simulink model "DataCenterStability"  (R2025b)
settings: Solver=daessc  StartTime=0  StopTime=7  FixedStep=5e-5  MaxStep=0.001  RelTol=1e-3
PostLoadFcn:
  | DataCenterParamScan
InitFcn:
  | opFile_ = fullfile(fileparts(which('DataCenterStability')), 'DataCenterStability_SteadyStateOP.mat');
  | if isfile(opFile_)
  |     tmp_ = load(opFile_, 'op');
  |     assignin('base', 'ssOP__', tmp_.op);
  | end
  | warning('off','physmod:common:mf:system:xform:DelayUnsupportedWithOperatingPoint');
  | warning('off','physmod:common:mf:system:xform:TimeUnsupportedWithOperatingPoint');
values from neighbouring files (symbols this model uses):
  baseVoltageDC = ups.Vdc    [DataCenterParamScan.m]
  bessConverterEfficiency = ups.DCBus.converterEff    [DataCenterParamScan.m]
  droopGain = ups.DCBus.droop    [DataCenterParamScan.m]
  filterInductance = ups.inverter.filterInductance    [DataCenterParamScan.m]
  filterInductanceAFE = ups.AFE.filterInductance    [DataCenterParamScan.m]
  filterResistance = ups.inverter.filterResistance    [DataCenterParamScan.m]
  filterResistanceAFE = ups.AFE.filterResistance    [DataCenterParamScan.m]
  frequency = ups.frequency    [DataCenterParamScan.m]
  G1 = 1    [DataCenterParamScan.m]
  G2 = 0    [DataCenterParamScan.m]
  iBatt = ups.batt.iRated    [DataCenterParamScan.m]
  initialMode = ups.batt.initialMode    [DataCenterParamScan.m]
  invKiId = ups.inverter.kiId    [DataCenterParamScan.m]
  invKiVd = ups.inverter.kiVd    [DataCenterParamScan.m]
  invKpId = ups.inverter.kpId    [DataCenterParamScan.m]
  invKpVd = ups.inverter.kpVd    [DataCenterParamScan.m]
  kpDC = ups.DCBus.kpDC    [DataCenterParamScan.m]
  N_pfc = round(N_total * [1/3, 1/3, 1/3])    [DataCenterParamScan.m]    (also in StabilityStudy.m = cfg.Topology.N_pfc)
  plantRating = ups.rating    [DataCenterParamScan.m]
  powerTau = 0.005    [DataCenterParamScan.m]
  rampRate = ups.batt.rampRate    [DataCenterParamScan.m]
  scan = obj.Cfg.GNC    [GNCAnalyzer.m]
  Ts = 5e-5    (= 5e-05)    [DataCenterParamScan.m]
  Vac = ups.Vac    [DataCenterParamScan.m]
  vBattMax = ups.batt.VMax    [DataCenterParamScan.m]
  vBattNom = ups.batt.Vnom    [DataCenterParamScan.m]
  vDCThreshold = ups.DCBus.VThreshold    [DataCenterParamScan.m]
  vGridMin = ups.DCBus.gridThreshold    [DataCenterParamScan.m]
undefined symbols (not defined in the file or in its folder): ctLimitDelayTime, DiscIntNeverNeededParam, ee_sli_rtmsupport, gcbh, itTray, pfc, serverTray, ups
libraries: fl_lib x77, nesl_utility x35, ee_lib x30, simulink x17, eeGeneralControl x14, datacenter_lib x12, eeTransforms x7, slpidlib x4, nesl_utility_internal x4, simulink_extras x3, datacenterCompositeLib x2, eePowerMeasurement x2
(part 4 of 5)

== system DataCenterStability/UPS/Rectifier/PFC Rectifier Controller ==
  VdcRef (V) : Inport
  QRef (pu) : Inport  Port=2
  VdcSens (V) : Inport  Port=3
  VabcSens (pu) : Inport  Port=4
  IabcSens (pu) : Inport  Port=5
  Reset : Inport  Port=6
  Current Controller : Subsystem
  DC Voltage Controller and Current Reference : Subsystem
  PLL : Subsystem
      settings: PortSchema="{\"entries\":[{\"content\":{\"sides\":[{\"content\":{\"connectorIds\":[\"Out1\",\"Out2\",\"Out3\",\"Out4\"]},\"type\":\"ConnectorPlacement.EquallySpacedRectSide\",\"uuid\":\"76485780-20fe-4fcf-8224-69648da6ed2a\"},{\"content\":{\"connectorIds\":[\"In1\"],\"side\":\"RIGHT\"},\"type\":\"ConnectorPlacement.EquallySpacedRectSide\",\"uuid\":\"f19a6390-e634-42c7-8d46-4cd80cbab182\"},{\"content\":{\"side\":\"TOP\"},\"type\":\"ConnectorPlacement.EquallySpacedRectSide\",\"uuid\":\"87682f72-1844-428e-be70-ad7ca3191ee3\"}]},\"type\":\"ConnectorPlacement.EquallySpacedConnector\",\"uuid\":\"f2136b07-48ec-402b-adb3-18c0bac2157c\"}],\"packageUris\":[\"http://schema.mathworks.com/mf0/Connector/R2020b\"],\"version\":\"1.0\"}"
  Rate Transition : RateTransition
  VabcRef (pu) : Outport
  Out Bus Element : Outport  Port=2  PortName=Visualization  Element=pllAngle [rad]
  Out Bus Element1 : Outport  Port=2  PortName=Visualization  Element=pllVmag [pu]
  Out Bus Element2 : Outport  Port=2  PortName=Visualization  Element=Idref [pu]
  Out Bus Element3 : Outport  Port=2  PortName=Visualization  Element=Iqref [pu]
  Out Bus Element5 : Outport  Port=2  PortName=Visualization  Element=IdCntrlError [pu]
  Out Bus Element6 : Outport  Port=2  PortName=Visualization  Element=IqCntrlError [pu]
  wires:
  Current Controller/3(IqCntrlError) -> Out Bus Element6/1
  Current Controller/2(IdCntrlError) -> Out Bus Element5/1
  PLL/1(theta) -> Out Bus Element/1, Current Controller/3(theta)
  Rate Transition/1 -> PLL/1(V)
  DC Voltage Controller and Current Reference/2(iqRef) -> Out Bus Element3/1, Current Controller/2(iqRef)
  DC Voltage Controller and Current Reference/1(idRef) -> Out Bus Element2/1, Current Controller/1(idRef)
  IabcSens (pu)/1 -> Current Controller/6(iabc(PU))
  PLL/3(Vq) -> Current Controller/5(vq)
  PLL/2(Vd) -> Current Controller/4(vd)
  VdcSens (V)/1 -> DC Voltage Controller and Current Reference/4(VdcSens)
  Current Controller/1(vabcRef) -> VabcRef (pu)/1
  PLL/4(mag) -> DC Voltage Controller and Current Reference/2(vPeak), Out Bus Element1/1
  QRef (pu)/1 -> DC Voltage Controller and Current Reference/1(qRef)
  VabcSens (pu)/1 -> Rate Transition/1
  VdcRef (V)/1 -> DC Voltage Controller and Current Reference/3(vdcRef)
  Reset/1 -> Current Controller/7(Reset), DC Voltage Controller and Current Reference/5(Reset)

== system DataCenterStability/UPS/Rectifier/Subsystem ==
  In : Inport
  Constant : Constant  Value=0  OutDataTypeStr=boolean
  Delay : Delay  DelayLength=700  InitialCondition=1  SampleTime=ups.sampleTime
  Detect Decrease : simulink/Logic and Bit Operations/Detect Decrease  vinit=0.0  OutDataTypeStr=boolean
  S-R Flip-Flop1 : simulink_extras/Flip Flops/S-R Flip-Flop  initial_condition=0
  Switch : Switch  Criteria=u2 > Threshold  SaturateOnIntegerOverflow=off  InputSameDT=off
  Out : Outport
  wires:
  In/1 -> Detect Decrease/1, Switch/3, Delay/1
  Switch/1 -> Out/1
  Detect Decrease/1 -> S-R Flip-Flop1/1
  Delay/1 -> Switch/1
  S-R Flip-Flop1/1 -> Switch/2
  Constant/1 -> S-R Flip-Flop1/2

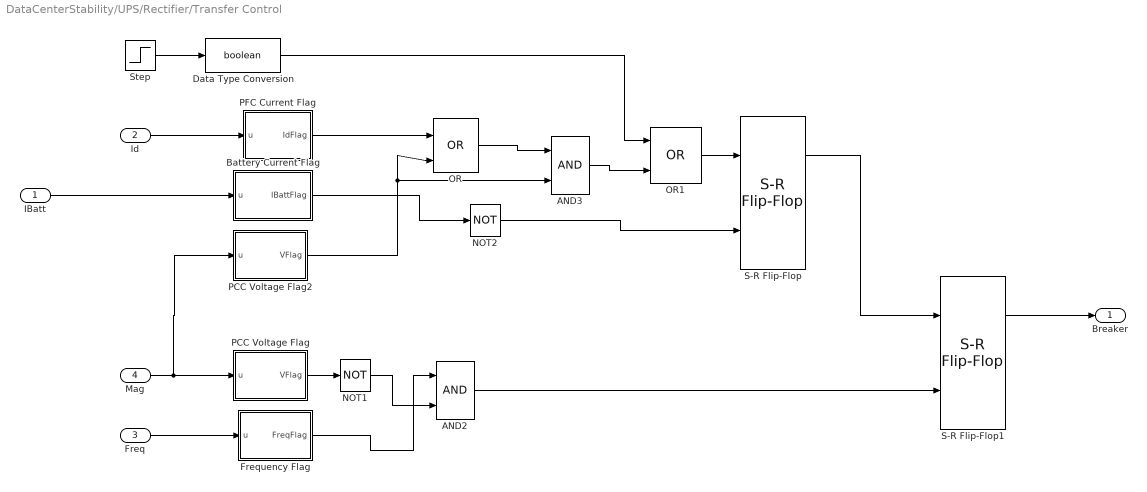
== system DataCenterStability/UPS/Rectifier/Transfer Control ==
  IBatt : Inport
  Id : Inport  Port=2
  Freq : Inport  Port=3
  Mag : Inport  Port=4
  AND2 : Logic  IconShape=distinctive  AllPortsSameDT=off  OutDataTypeStr=boolean
  AND3 : Logic  IconShape=distinctive  AllPortsSameDT=off  OutDataTypeStr=boolean
  Battery Current Flag : Subsystem
  Data Type Conversion : DataTypeConversion  OutDataTypeStr=boolean  SaturateOnIntegerOverflow=off  RndMeth=Floor
  Frequency Flag : Subsystem
  NOT1 : Logic  Operator=NOT  IconShape=distinctive  AllPortsSameDT=off  OutDataTypeStr=boolean
  NOT2 : Logic  Operator=NOT  IconShape=distinctive  AllPortsSameDT=off  OutDataTypeStr=boolean
  OR : Logic  Operator=OR  IconShape=distinctive  AllPortsSameDT=off  OutDataTypeStr=boolean
  OR1 : Logic  Operator=OR  IconShape=distinctive  AllPortsSameDT=off  OutDataTypeStr=boolean
  PCC Voltage Flag : Subsystem
  PCC Voltage Flag2 : Subsystem
  PFC Current Flag : Subsystem
  S-R Flip-Flop : simulink_extras/Flip Flops/S-R Flip-Flop  initial_condition=0
  S-R Flip-Flop1 : simulink_extras/Flip Flops/S-R Flip-Flop  initial_condition=0
  Step : Step  Time=0  SampleTime=0
  Breaker : Outport
  wires:
  PFC Current Flag/1(IdFlag) -> OR/1
  S-R Flip-Flop/1 -> S-R Flip-Flop1/1
  Id/1 -> PFC Current Flag/1(u)
  Mag/1 -> PCC Voltage Flag2/1(u), PCC Voltage Flag/1(u)
  Freq/1 -> Frequency Flag/1(u)
  S-R Flip-Flop1/1 -> Breaker/1
  IBatt/1 -> Battery Current Flag/1(u)
  Frequency Flag/1(FreqFlag) -> AND2/1
  NOT2/1 -> S-R Flip-Flop/2
  Battery Current Flag/1(IBattFlag) -> NOT2/1
  AND2/1 -> S-R Flip-Flop1/2
  OR/1 -> AND3/1
  Step/1 -> Data Type Conversion/1
  AND3/1 -> OR1/2
  Data Type Conversion/1 -> OR1/1
  OR1/1 -> S-R Flip-Flop/1
  PCC Voltage Flag/1(VFlag) -> NOT1/1
  NOT1/1 -> AND2/2
  PCC Voltage Flag2/1(VFlag) -> AND3/2, OR/2

== system DataCenterStability/UPS/DC-Link/BESS/DC-DC Converter Controller ==
  Voref : Inport
  Vo : Inport  Port=2
  vBatt : Inport  Port=3
  iPFC : Inport  Port=4
  iCharge : Inport  Port=5
  iBatt : Inport  Port=6
  vPCC : Inport  Port=7
  Breaker : Inport  Port=8
  Current Reference Generator : Subsystem
  Gain : Gain  Gain=iBatt+4000
  Mode Control : Subsystem
  Saturation : Saturate  UpperLimit=iBatt  LowerLimit=-iBatt
  Simulink-PS Converter : nesl_utility/Simulink-PS Converter  PhysicalDomain=network_engine_domain  SubClassName=ps_input  LeftPortType=input  RightPortType=output  PseudoPeriodic=off  Frequencies=[]  NoiseDistribution=none  NoiseParameters=[]  Unit=1  AffineConversion=off  FilteringAndDerivatives=provide  SimscapeFilterOrder=1  InputFilterTimeConstant=0.001  UdotUserProvided=0
  Terminator1 : Terminator
  mod : PMIOPort  Side=Right
  wires:
  Gain/1 -> Saturation/1
  iPFC/1 -> Mode Control/1(iPFC)
  vBatt/1 -> Mode Control/3(vBatt)
  Current Reference Generator/1(i) -> Gain/1
  Mode Control/1(DischargeFlag) -> Current Reference Generator/2(DischargeFlag)
  Saturation/1 -> Simulink-PS Converter/1
  iBatt/1 -> Mode Control/7(iBatt)
  vPCC/1 -> Mode Control/4(vPCC)
  Breaker/1 -> Mode Control/5(Breaker)
  iCharge/1 -> Mode Control/6(iCharg)
  Vo/1 -> Mode Control/2(Vdc)
  Mode Control/3(iRef) -> Current Reference Generator/4(I)
  Mode Control/5(Mode) -> Terminator1/1
  Voref/1 -> Current Reference Generator/1(VoRef)
  Mode Control/2(vOut) -> Current Reference Generator/3(Vo)
  Mode Control/4(droopMode) -> Current Reference Generator/5(Mode)
  connections:
  mod/RConn1 -- Simulink-PS Converter/RConn1

== system DataCenterStability/UPS/Inverter/Filter & Measurements/ Measurements ==
  V : Inport
  I : Inport  Port=2
  w : Inport  Port=3
  Theta : Inport  Port=4
  Measurement1 : Subsystem
  Measurement2 : Subsystem
  Subsystem : Subsystem
  Out Bus Element : Outport  PortName=VIbus  Element=Vq
  Out Bus Element1 : Outport  PortName=VIbus  Element=Vd
  Out Bus Element2 : Outport  PortName=VIbus  Element=Freq
  Out Bus Element3 : Outport  PortName=VIbus  Element=Theta
  Out Bus Element4 : Outport  PortName=VIbus  Element=Vmag
  Out Bus Element5 : Outport  PortName=VIbus  Element=Iq
  Out Bus Element6 : Outport  PortName=VIbus  Element=Id
  Out Bus Element7 : Outport  PortName=VIbus  Element=Iabc
  Out Bus Element8 : Outport  PortName=VIbus  Element=Vabc
  wires:
  Subsystem/6(Id1) -> Out Bus Element6/1
  Subsystem/7(Iq1) -> Out Bus Element5/1
  Measurement1/1(Vg) -> Subsystem/2(Iabc), Out Bus Element7/1
  I/1 -> Measurement1/1(u)
  Measurement2/1(Vg) -> Subsystem/1(Vabc), Out Bus Element8/1
  Subsystem/4(Vd) -> Out Bus Element1/1
  Subsystem/5(Vq) -> Out Bus Element/1
  V/1 -> Measurement2/1(u)
  w/1 -> Subsystem/3(w)
  Theta/1 -> Subsystem/4(Theta)
  Subsystem/1(mag) -> Out Bus Element4/1
  Subsystem/2(freq) -> Out Bus Element2/1
  Subsystem/3(angle) -> Out Bus Element3/1

== system DataCenterStability/UPS/Inverter/Inverter Controller/Current Limiter ==
  BusElementIn : Inport  PortName=VI  Element=Id
  BusElementIn1 : Inport  PortName=VI  Element=Iq
  Vd : Inport  Port=2
  Vq : Inport  Port=3
  Add : Sum  Inputs=+-
  Add1 : Sum  Inputs=+-
  Current Limiter : Subsystem  Variant=on  VariantControlMode=label  VariantControl=Choice  LabelModeActiveChoice=Virtual Impedance
  VdRef : Outport
  VqRef : Outport  Port=2
  Idmax : Outport  Port=3
  Iqmax : Outport  Port=4
  wires:
  BusElementIn/1 -> Current Limiter/1(Igd)
  BusElementIn1/1 -> Current Limiter/2(Igq)
  Current Limiter/3(Idmax) -> Idmax/1
  Current Limiter/4(Iqmax) -> Iqmax/1
  Current Limiter/1(delVd) -> Add/2
  Vd/1 -> Add/1
  Add1/1 -> VqRef/1
  Current Limiter/2(delVq) -> Add1/2
  Vq/1 -> Add1/1
  Add/1 -> VdRef/1

== system DataCenterStability/UPS/Inverter/Inverter Controller/Droop Control ==
  note: Vs-delV
  Add : Sum  Inputs=+-
  Constant1 : Constant  Value=powerFreq*2*pi
  Constant2 : Constant  Value=0
  Constant3 : Constant
  Constant4 : Constant  Value=0
  Constant5 : Constant  Value=pi/2
  Integrator with Wrapped State (Discrete or Continuous) : eeGeneralControl/Integrator with Wrapped State (Discrete or Continuous)  LabelModeActiveChoice=Discrete  WrappedStateUpperValue=pi  WrappedStateLowerValue=-pi  x0=0  Ts=Ts
  Saturation : Saturate  UpperLimit=1.5  LowerLimit=0.9
  Sum1 : Sum  Inputs=|++
  Vdref : Outport
  Vqref : Outport  Port=2
  omega : Outport  Port=3
  Theta : Outport  Port=4
  wires:
  Constant1/1 -> Integrator with Wrapped State (Discrete or Continuous)/1, omega/1
  Sum1/1 -> Saturation/1  "V"
  Constant5/1 -> Add/2
  Constant3/1 -> Sum1/1
  Saturation/1 -> Vdref/1
  Integrator with Wrapped State (Discrete or Continuous)/1 -> Add/1
  Add/1 -> Theta/1
  Constant4/1 -> Vqref/1
  Constant2/1 -> Sum1/2

== system DataCenterStability/UPS/Inverter/Inverter Controller/VoltageCurrentControl ==
  BusElementIn : Inport  PortName=measure  Element=Vq
  BusElementIn1 : Inport  PortName=measure  Element=Vd
  BusElementIn2 : Inport  PortName=measure  Element=Iq
  BusElementIn3 : Inport  PortName=measure  Element=Id
  Vdref : Inport  Port=2
  Vqref : Inport  Port=3
  Idmax : Inport  Port=4
  Iqmax : Inport  Port=5
  w : Inport  Port=6
  Angle : Inport  Port=7
  Controller : Subsystem
  Modulation Signal : Subsystem
  mabc : Outport
  wires:
  Vdref/1 -> Controller/2(Vdref)
  Controller/1(Vd) -> Modulation Signal/1(Vd)
  Modulation Signal/1(mabc) -> mabc/1
  Controller/2(Vq) -> Modulation Signal/2(Vq)
  w/1 -> Controller/1(Angfreq)
  Angle/1 -> Modulation Signal/3(Angle)
  BusElementIn/1 -> Controller/5(Vsq)
  BusElementIn1/1 -> Controller/4(Vsd)
  BusElementIn2/1 -> Controller/7(Iq)
  BusElementIn3/1 -> Controller/6(Id)
  Vqref/1 -> Controller/3(Vqref)
  Idmax/1 -> Controller/8(IqMax)
  Iqmax/1 -> Controller/9(IdMax)

== system DataCenterStability/UPS/Rectifier/Filter & AC measurements/Current ==
  Isabc : Inport
  Demux : Demux  Outputs=3
  Mux : Mux  Inputs=3
  Unit Delay : UnitDelay  SampleTime=-1
  Iabc : Outport
  wires:
  Mux/1 -> Iabc/1
  Unit Delay/1 -> Demux/1
  Isabc/1 -> Unit Delay/1
  Demux/1 -> Mux/1
  Demux/2 -> Mux/2
  Demux/3 -> Mux/3

== system DataCenterStability/UPS/Rectifier/Filter & AC measurements/PLL ==
  Iabc : Inport
  V : Inport  Port=2
  Constant1 : Constant  Value=pi/2  SampleTime=Ts
  Data Type Conversion Inherited : simulink/Signal Attributes/Data Type Conversion Inherited  ConvertRealWorld=Real World Value  DoSatur=off
  Demux : Demux  Outputs=3
  Park Transform : eeTransforms/Park Transform  AxisAlignment=D-axis  PowerInvariant=off
  "Sinusoidal Measurement (PLL, Three-Phase)" : eeSinusoidalMeasurementV2/Sinusoidal Measurement (PLL, Three-Phase)  InputFilter=on  InputNormalization=off  Kp_LF=ups.AFE.kpPLL  Ki_LF=ups.AFE.kiPLL  F0=frequency  Theta0=0  Ts=Ts
  Sum : Sum  Inputs=|+-
  Terminator : Terminator
  Terminator2 : Terminator
  Id : Outport
  freq : Outport  Port=2
  mag : Outport  Port=3
  wires:
  Data Type Conversion Inherited/1 -> Sum/2
  Constant1/1 -> Data Type Conversion Inherited/2
  V/1 -> "Sinusoidal Measurement (PLL, Three-Phase)"/1
  "Sinusoidal Measurement (PLL, Three-Phase)"/2 -> Sum/1, Data Type Conversion Inherited/1
  Park Transform/1 -> Demux/1
  Demux/3 -> Terminator/1
  Sum/1 -> Park Transform/2
  Demux/1 -> Id/1
  "Sinusoidal Measurement (PLL, Three-Phase)"/1 -> freq/1
  Iabc/1 -> Park Transform/1
  Demux/2 -> Terminator2/1
  "Sinusoidal Measurement (PLL, Three-Phase)"/3 -> mag/1

== system DataCenterStability/UPS/Rectifier/Filter & AC measurements/Voltage ==
  Vsabc : Inport
  Demux1 : Demux  Outputs=3
  Mux1 : Mux  Inputs=3
  Unit Delay : UnitDelay  SampleTime=-1
  Vabc : Outport
  wires:
  Mux1/1 -> Vabc/1
  Unit Delay/1 -> Demux1/1
  Vsabc/1 -> Unit Delay/1
  Demux1/1 -> Mux1/1
  Demux1/2 -> Mux1/2
  Demux1/3 -> Mux1/3

== system DataCenterStability/UPS/Rectifier/PFC Rectifier Controller/Current Controller ==
  idRef : Inport
  iqRef : Inport  Port=2
  theta : Inport  Port=3
  vd : Inport  Port=4
  vq : Inport  Port=5
  iabc(PU) : Inport  Port=6
  Reset : Inport  Port=7
  Demux1 : Demux  Outputs=3
  Id and Iq Controller : Subsystem
  Inverse Park Transform : eeTransforms/Inverse Park Transform  AxisAlignment=D-axis  PowerInvariant=off
  Park Transform : eeTransforms/Park Transform  AxisAlignment=D-axis  PowerInvariant=off
  Saturation : Saturate  UpperLimit=1.5  LowerLimit=-1.5
  Terminator1 : Terminator
  vabcRef : Outport
  IdCntrlError : Outport  Port=2
  IqCntrlError : Outport  Port=3
  wires:
  Id and Iq Controller/2(IdCntrlError) -> IdCntrlError/1
  Id and Iq Controller/3(IqCntrlError) -> IqCntrlError/1
  Id and Iq Controller/1(vdqoRef) -> Inverse Park Transform/1
  vq/1 -> Id and Iq Controller/6(vq)
  Demux1/2 -> Id and Iq Controller/4(iqSens)  "iqSens"
  iqRef/1 -> Id and Iq Controller/2(iqRef)
  Demux1/1 -> Id and Iq Controller/3(IdSens)  "IdSens"
  idRef/1 -> Id and Iq Controller/1(idRef)
  vd/1 -> Id and Iq Controller/5(vd)
  Inverse Park Transform/1 -> Saturation/1
  iabc(PU)/1 -> Park Transform/1
  theta/1 -> Park Transform/2, Inverse Park Transform/2
  Demux1/3 -> Terminator1/1
  Park Transform/1 -> Demux1/1
  Saturation/1 -> vabcRef/1
  Reset/1 -> Id and Iq Controller/7(Reset)

== system DataCenterStability/UPS/Rectifier/PFC Rectifier Controller/DC Voltage Controller and Current Reference ==
  qRef : Inport
  vPeak : Inport  Port=2
  vdcRef : Inport  Port=3
  VdcSens : Inport  Port=4
  Reset : Inport  Port=5
  Constant : Constant  SampleTime=Ts
  Data Type Conversion Inherited : simulink/Signal Attributes/Data Type Conversion Inherited  ConvertRealWorld=Real World Value  DoSatur=off
  Gain : Gain  Gain=-1
  Iq Reference : Subsystem
  Switch : Switch  Criteria=u2 > Threshold  SaturateOnIntegerOverflow=off  InputSameDT=off
  Voltage Controller : Subsystem
  idRef : Outport
  iqRef : Outport  Port=2
  wires:
  Constant/1 -> Data Type Conversion Inherited/2
  Data Type Conversion Inherited/1 -> Switch/3
  Gain/1 -> iqRef/1
  qRef/1 -> Iq Reference/2(Q_ref)
  Voltage Controller/1(Id) -> idRef/1
  vdcRef/1 -> Voltage Controller/1(Vdcref)
  VdcSens/1 -> Voltage Controller/2(Vdcmeas)
  Iq Reference/1(iq_ref) -> Gain/1
  vPeak/1 -> Switch/2, Switch/1, Data Type Conversion Inherited/1
  Switch/1 -> Iq Reference/1(V_mag)
  Reset/1 -> Voltage Controller/3(Reset)

== system DataCenterStability/UPS/Rectifier/PFC Rectifier Controller/PLL ==
  V : Inport
  Constant1 : Constant  Value=pi/2  SampleTime=Ts
  Data Type Conversion Inherited : simulink/Signal Attributes/Data Type Conversion Inherited  ConvertRealWorld=Real World Value  DoSatur=off
  Demux : Demux  Outputs=3
  Park Transform : eeTransforms/Park Transform  AxisAlignment=D-axis  PowerInvariant=off
  "Sinusoidal Measurement (PLL, Three-Phase)" : eeSinusoidalMeasurementV2/Sinusoidal Measurement (PLL, Three-Phase)  InputFilter=on  InputNormalization=off  Kp_LF=KpPLL  Ki_LF=KiPLL  F0=Freq  Theta0=0  Ts=Ts
  Sum : Sum  Inputs=|+-
  Terminator : Terminator
  Terminator1 : Terminator
  theta : Outport
  Vd : Outport  Port=2
  Vq : Outport  Port=3
  mag : Outport  Port=4
  wires:
  Data Type Conversion Inherited/1 -> Sum/2
  Constant1/1 -> Data Type Conversion Inherited/2
  V/1 -> Park Transform/1, "Sinusoidal Measurement (PLL, Three-Phase)"/1
  "Sinusoidal Measurement (PLL, Three-Phase)"/2 -> Sum/1, Data Type Conversion Inherited/1
  Park Transform/1 -> Demux/1
  Demux/3 -> Terminator/1
  "Sinusoidal Measurement (PLL, Three-Phase)"/3 -> mag/1
  Sum/1 -> Park Transform/2, theta/1
  Demux/2 -> Vq/1
  Demux/1 -> Vd/1
  "Sinusoidal Measurement (PLL, Three-Phase)"/1 -> Terminator1/1

== system DataCenterStability/UPS/Rectifier/Transfer Control/Battery Current Flag ==
  u : Inport
  AND : Logic  IconShape=distinctive  AllPortsSameDT=off  OutDataTypeStr=boolean
  Compare To Constant : simulink/Logic and Bit Operations/Compare To Constant  relop=>=  const=0.04  OutDataTypeStr=boolean
  Compare To Constant1 : simulink/Logic and Bit Operations/Compare To Constant  relop=<=  const=-10  OutDataTypeStr=boolean
  Data Type Conversion : DataTypeConversion  SaturateOnIntegerOverflow=off  RndMeth=Floor
  Data Type Conversion1 : DataTypeConversion  OutDataTypeStr=double  SaturateOnIntegerOverflow=off  RndMeth=Floor
  Discrete-Time Integrator : DiscreteIntegrator  IntegratorMethod=Integration: Backward Euler  ExternalReset=falling  SampleTime=ups.sampleTime  LimitOutput=on  UpperSaturationLimit=0.04  LowerSaturationLimit=0  ICPrevOutput=DiscIntNeverNeededParam  ICPrevScaledInput=DiscIntNeverNeededParam
  Scope : Scope  NumInputPorts=2
      settings: ActiveDisplayYMinimum=-1  ActiveDisplayYMaximum=1  DataLoggingVariableName=ScopeData51
  Scope1 : Scope
      settings: ActiveDisplayYMinimum=-1  ActiveDisplayYMaximum=1  DataLoggingVariableName=ScopeData52
  Scope2 : Scope
      settings: ActiveDisplayYMinimum=-1  ActiveDisplayYMaximum=1  DataLoggingVariableName=ScopeData54
  IBattFlag : Outport
  wires:
  AND/1 -> Data Type Conversion/1
  Compare To Constant1/1 -> Data Type Conversion1/1
  Compare To Constant/1 -> AND/2
  u/1 -> Scope2/1, Compare To Constant1/1
  Discrete-Time Integrator/1 -> Scope/2, Compare To Constant/1
  Data Type Conversion/1 -> Scope1/1, IBattFlag/1
  Data Type Conversion1/1 -> Discrete-Time Integrator/1, Scope/1, AND/1, Discrete-Time Integrator/2

== system DataCenterStability/UPS/Rectifier/Transfer Control/Frequency Flag ==
  u : Inport
  AND : Logic  IconShape=distinctive  AllPortsSameDT=off  OutDataTypeStr=boolean
  Abs : Abs  SaturateOnIntegerOverflow=off
  Add : Sum  Inputs=+-
  Compare To Constant : simulink/Logic and Bit Operations/Compare To Constant  relop=>  const=0.5  OutDataTypeStr=boolean
  Compare To Constant1 : simulink/Logic and Bit Operations/Compare To Constant  relop=<=  const=0.01*frequency  OutDataTypeStr=boolean
  Constant : Constant  Value=frequency
  Data Type Conversion : DataTypeConversion  SaturateOnIntegerOverflow=off  RndMeth=Floor
  Data Type Conversion1 : DataTypeConversion  OutDataTypeStr=double  SaturateOnIntegerOverflow=off  RndMeth=Floor
  Discrete-Time Integrator : DiscreteIntegrator  IntegratorMethod=Integration: Backward Euler  ExternalReset=falling  SampleTime=ups.sampleTime  LimitOutput=on  UpperSaturationLimit=0.6  LowerSaturationLimit=0  ICPrevOutput=DiscIntNeverNeededParam  ICPrevScaledInput=DiscIntNeverNeededParam
  FreqFlag : Outport
  wires:
  AND/1 -> Data Type Conversion/1
  Compare To Constant/1 -> AND/2
  Discrete-Time Integrator/1 -> Compare To Constant/1
  Data Type Conversion/1 -> FreqFlag/1
  Data Type Conversion1/1 -> Discrete-Time Integrator/1, AND/1, Discrete-Time Integrator/2
  u/1 -> Add/1
  Constant/1 -> Add/2
  Add/1 -> Abs/1
  Abs/1 -> Compare To Constant1/1
  Compare To Constant1/1 -> Data Type Conversion1/1

== system DataCenterStability/UPS/Rectifier/Transfer Control/PCC Voltage Flag ==
  u : Inport
  AND : Logic  IconShape=distinctive  AllPortsSameDT=off  OutDataTypeStr=boolean
  Abs : Abs  SaturateOnIntegerOverflow=off
  Add : Sum  Inputs=+-
  Compare To Constant : simulink/Logic and Bit Operations/Compare To Constant  relop=>  const=0.2  OutDataTypeStr=boolean
  Compare To Constant1 : simulink/Logic and Bit Operations/Compare To Constant  relop=>=  const=0.1  OutDataTypeStr=boolean
  Constant : Constant
  Data Type Conversion : DataTypeConversion  SaturateOnIntegerOverflow=off  RndMeth=Floor
  Data Type Conversion1 : DataTypeConversion  OutDataTypeStr=double  SaturateOnIntegerOverflow=off  RndMeth=Floor
  Discrete-Time Integrator : DiscreteIntegrator  IntegratorMethod=Integration: Backward Euler  ExternalReset=falling  SampleTime=ups.sampleTime  LimitOutput=on  UpperSaturationLimit=0.6  LowerSaturationLimit=0  ICPrevOutput=DiscIntNeverNeededParam  ICPrevScaledInput=DiscIntNeverNeededParam
  VFlag : Outport
  wires:
  AND/1 -> Data Type Conversion/1
  Compare To Constant/1 -> AND/2
  Discrete-Time Integrator/1 -> Compare To Constant/1
  Data Type Conversion/1 -> VFlag/1
  Data Type Conversion1/1 -> Discrete-Time Integrator/1, AND/1, Discrete-Time Integrator/2
  u/1 -> Add/1
  Constant/1 -> Add/2
  Add/1 -> Abs/1
  Compare To Constant1/1 -> Data Type Conversion1/1
  Abs/1 -> Compare To Constant1/1

== system DataCenterStability/UPS/Rectifier/Transfer Control/PCC Voltage Flag2 ==
  u : Inport
  AND : Logic  IconShape=distinctive  AllPortsSameDT=off  OutDataTypeStr=boolean
  Abs : Abs  SaturateOnIntegerOverflow=off
  Add : Sum  Inputs=+-
  Compare To Constant : simulink/Logic and Bit Operations/Compare To Constant  relop=>  const=0.15  OutDataTypeStr=boolean
  Compare To Constant1 : simulink/Logic and Bit Operations/Compare To Constant  relop=>=  const=0.9  OutDataTypeStr=boolean
  Constant : Constant
  Data Type Conversion : DataTypeConversion  SaturateOnIntegerOverflow=off  RndMeth=Floor
  Data Type Conversion1 : DataTypeConversion  OutDataTypeStr=double  SaturateOnIntegerOverflow=off  RndMeth=Floor
  Discrete-Time Integrator : DiscreteIntegrator  IntegratorMethod=Integration: Backward Euler  ExternalReset=falling  SampleTime=ups.sampleTime  LimitOutput=on  UpperSaturationLimit=4  LowerSaturationLimit=0  ICPrevOutput=DiscIntNeverNeededParam  ICPrevScaledInput=DiscIntNeverNeededParam
  VFlag : Outport
  wires:
  AND/1 -> Data Type Conversion/1
  Compare To Constant/1 -> AND/2
  Discrete-Time Integrator/1 -> Compare To Constant/1
  Data Type Conversion/1 -> VFlag/1
  Data Type Conversion1/1 -> Discrete-Time Integrator/1, AND/1, Discrete-Time Integrator/2
  u/1 -> Add/1
  Constant/1 -> Add/2
  Add/1 -> Abs/1
  Compare To Constant1/1 -> Data Type Conversion1/1
  Abs/1 -> Compare To Constant1/1

== system DataCenterStability/UPS/Rectifier/Transfer Control/PFC Current Flag ==
  u : Inport
  AND : Logic  IconShape=distinctive  AllPortsSameDT=off  OutDataTypeStr=boolean
  Compare To Constant : simulink/Logic and Bit Operations/Compare To Constant  relop=>  const=0.02  OutDataTypeStr=boolean
  Compare To Constant1 : simulink/Logic and Bit Operations/Compare To Constant  relop=<=  const=0.01  OutDataTypeStr=boolean
  Data Type Conversion : DataTypeConversion  SaturateOnIntegerOverflow=off  RndMeth=Floor
  Data Type Conversion1 : DataTypeConversion  OutDataTypeStr=double  SaturateOnIntegerOverflow=off  RndMeth=Floor
  Discrete-Time Integrator : DiscreteIntegrator  IntegratorMethod=Integration: Backward Euler  ExternalReset=falling  SampleTime=ups.sampleTime  LimitOutput=on  UpperSaturationLimit=0.04  LowerSaturationLimit=0  ICPrevOutput=DiscIntNeverNeededParam  ICPrevScaledInput=DiscIntNeverNeededParam
  Scope : Scope  NumInputPorts=2
      settings: ActiveDisplayYMinimum=-1  ActiveDisplayYMaximum=1  DataLoggingVariableName=ScopeData49
  Scope1 : Scope
      settings: ActiveDisplayYMinimum=-1  ActiveDisplayYMaximum=1  DataLoggingVariableName=ScopeData50
  IdFlag : Outport
  wires:
  AND/1 -> Data Type Conversion/1
  Compare To Constant1/1 -> Data Type Conversion1/1
  Compare To Constant/1 -> Scope/2, AND/2
  u/1 -> Compare To Constant1/1
  Discrete-Time Integrator/1 -> Scope1/1, Compare To Constant/1
  Data Type Conversion/1 -> IdFlag/1
  Data Type Conversion1/1 -> Scope/1, Discrete-Time Integrator/1, AND/1, Discrete-Time Integrator/2

== system DataCenterStability/UPS/DC-Link/BESS/DC-DC Converter Controller/Current Reference Generator ==
  VoRef : Inport
  DischargeFlag : Inport  Port=2
  Vo : Inport  Port=3
  I : Inport  Port=4
  Mode : Inport  Port=5
  Add : Sum  Inputs=-+
  Gain : Gain  Gain=droopGain
  Low-Pass Filter (Discrete or Continuous) : eeGeneralControl/Low-Pass Filter (Discrete or Continuous)  K=1  T=0.001  B=inf  A=-inf  init_option=Inherited from block input  x0=0  Ts=-1
  PID Controller : slpidlib/PID Controller  Controller=PI  Form=Parallel  TimeDomain=Discrete-time  UseExternalTs=off  SampleTime=-1  IntegratorMethod=Forward Euler  FilterMethod=Forward Euler  ControllerParametersSource=internal  P=kpDC%500  I=kiDC%500  UseKiTs=off  D=0  UseExternalDerivativeSource=off  N=100  UseFilter=on  TunerSelectOption=Transfer Function Based (PID Tuner App)  InitialConditionSource=internal  InitialConditionForIntegrator=0  InitialConditionForFilter=0  DifferentiatorICPrevScaledInput=0  ExternalReset=rising  TrackingMode=off  Kt=1  LimitOutput=on  SatLimitsSource=internal  UpperSaturationLimit=0  LowerSaturationLimit=-5  LinearizeAsGain=on  AntiWindupMode=clamping  Kb=1  LimitIntegrator=off  UpperIntegratorSaturationLimit=4  LowerIntegratorSaturationLimit=-4  POutMin=[]  POutMax=[]  IOutMin=[]  IOutMax=[]  DOutMin=[]  DOutMax=[]  NOutMin=[]  NOutMax=[]  SumOutMin=[]  SumOutMax=[]  SaturationOutMin=[]  SaturationOutMax=[]  PParamMin=[]  PParamMax=[]  IParamMin=[]  IParamMax=[]  DParamMin=[]  DParamMax=[]  NParamMin=[]  NParamMax=[]  KbParamMin=[]  KbParamMax=[]  KtParamMin=[]  KtParamMax=[]  KbOutMin=[]  KbOutMax=[]  KtOutMin=[]  KtOutMax=[]  IntegratorOutMin=[]  IntegratorOutMax=[]  FilterOutMin=[]  FilterOutMax=[]  SumI1OutMin=[]  SumI1OutMax=[]  SumI2OutMin=[]  SumI2OutMax=[]  SumI3OutMin=[]  SumI3OutMax=[]  SumI4OutMin=[]  SumI4OutMax=[]  SumDOutMin=[]  SumDOutMax=[]  DifferentiatorOutMin=[]  DifferentiatorOutMax=[]  FilterDiffOutCoefMin=[]  FilterDiffOutCoefMax=[]  ReciprocalOutMin=[]  ReciprocalOutMax=[]  SumDenOutMin=[]  SumDenOutMax=[]  SumNumOutMin=[]  SumNumOutMax=[]  DivideOutMin=[]  DivideOutMax=[]  UdiffTsProdOutMin=[]  UdiffTsProdOutMax=[]  NTsProdOutMin=[]  NTsProdOutMax=[]  UintegralTsProdOutMin=[]  UintegralTsProdOutMax=[]  UngainTsProdOutMin=[]  UngainTsProdOutMax=[]  ClampingZeroOutDataTypeStr=Inherit: Inherit via back propagation  ClampingZeroOutMin=[]  ClampingZeroOutMax=[]  FilterDenConstantOutDataTypeStr=Inherit: Inherit via back propagation  FilterDenConstantOutMin=[]  FilterDenConstantOutMax=[]  PCopyOutDataTypeStr=Inherit: Inherit via back propagation  PCopyOutMin=[]  PCopyOutMax=[]  NCopyOutDataTypeStr=Inherit: Inherit via back propagation  NCopyOutMin=[]  NCopyOutMax=[]  IntegratorContinuousStateAttributes=''  IntegratorStateMustResolveToSignalObject=off  IntegratorRTWStateStorageClass=Auto  FilterContinuousStateAttributes=''  FilterStateMustResolveToSignalObject=off  FilterRTWStateStorageClass=Auto  ParallelPVariant=InternalParameters  IdealPVariant=Disabled  IVariant=InternalParameters  DVariant=Disabled  IntegratorVariant=Discrete  SatVariant=Enabled  AWVariant=DiscClampingParallel  PCopyVariant=Disabled  TRVariant=Disabled  FdbkBlocksVariant=Forward  IdealPFdbkVariant=Disabled  SatFdbkVariant=Disabled  DerivativeFilterVariant=Disabled  NVariant=Disabled  NCopyVariant=Disabled_SignalSpec  FilterICVariant=Disabled  IntegratorICVariant=InternalICs  ExternalResetVariant=ExternalReset  TRSumVariant=Passthrough  SumFdbkVariant=Disabled  SumVariant=Sum_PI  TsampFilterVariant=InternalTs  TsampNgainVariant=Passthrough  TsampIntegralVariant=Disabled_SignalSpec  ExternalSaturationOutDataTypeStr=Inherit: Same as second input  DerivativeSourceVariant=Disabled  PreIntVariant=InternalPreInt
  Saturation1 : Saturate  UpperLimit=0  LowerLimit=-10
  Switch1 : Switch  Criteria=u2 > Threshold  SaturateOnIntegerOverflow=off  InputSameDT=off
  Switch3 : Switch  Criteria=u2 > Threshold  SaturateOnIntegerOverflow=off  InputSameDT=off
  i : Outport  VectorParamsAs1DForOutWhenUnconnected=off
  wires:
  Switch1/1 -> Low-Pass Filter (Discrete or Continuous)/1
  Low-Pass Filter (Discrete or Continuous)/1 -> i/1
  Gain/1 -> Saturation1/1
  Switch3/1 -> Switch1/1
  Add/1 -> PID Controller/1, Gain/1
  VoRef/1 -> Add/1
  Vo/1 -> Add/2
  DischargeFlag/1 -> PID Controller/2, Switch1/2
  Mode/1 -> Switch3/2
  Saturation1/1 -> Switch3/1
  PID Controller/1 -> Switch3/3
  I/1 -> Switch1/3

== system DataCenterStability/UPS/DC-Link/BESS/DC-DC Converter Controller/Mode Control ==
  iPFC : Inport
  Vdc : Inport  Port=2
  vBatt : Inport  Port=3
  vPCC : Inport  Port=4
  Breaker : Inport  Port=5
  iCharg : Inport  Port=6
  iBatt : Inport  Port=7
  BMS : Stateflow chart  TreatAsAtomicUnit=on  mask(Microgrid Transition and Dispatch Control){VMaxBatt=vBattMax, VdcRated=baseVoltageDC, iThreshold=vGridMin, iBattTh=10, vThreshold=0.9, VMaxDC=vDCThreshold, VBattNom=vBattMax, initialMode=initialMode}
      mask prompts: VMaxBatt "Maximum Battery Voltage (V)"; VdcRated "Rated DC bus voltage (V)"; iThreshold "Threshold mains current (A)"; iBattTh "Threshold battery current (A)"; vThreshold "Threshold mains voltage (V)"; VMaxDC "Threshold DC Bus Voltage (V)"; VBattNom "Battery nominal voltage (V)"; initialMode "Initial Operating Mode"
      mask help: This subsystem implements the transitions and the corresponding dispatch functions in the microgrid
  Compare To Constant : simulink/Logic and Bit Operations/Compare To Constant  relop===  const=4  OutDataTypeStr=boolean
  Constant : Constant  Value=0.98  OutDataTypeStr=double
  DischargeFlag : Outport
  vOut : Outport  Port=2
  iRef : Outport  Port=3
  droopMode : Outport  Port=4
  Mode : Outport  Port=5
  wires:
  iPFC/1 -> BMS/1(iPFC)
  Vdc/1 -> BMS/2(Vdc)
  vBatt/1 -> BMS/3(VBatt)
  Compare To Constant/1 -> DischargeFlag/1
  Constant/1 -> BMS/4(SOC)
  Breaker/1 -> BMS/5(breakerStatus)
  BMS/1(mode) -> Compare To Constant/1, Mode/1
  vPCC/1 -> BMS/6(VPCC)
  iCharg/1 -> BMS/7(iCharg)
  BMS/3(vOut) -> vOut/1
  BMS/2(iRef) -> iRef/1
  iBatt/1 -> BMS/8(iBatt)
  BMS/4(droopMode) -> droopMode/1

== system DataCenterStability/UPS/Inverter/Filter & Measurements/ Measurements/Measurement1 ==
  u : Inport
  Lead-Lag (Discrete or Continuous) : eeGeneralControl/Lead-Lag (Discrete or Continuous)  T1=0  T2=1e-3  B=inf  A=-inf  init_option=Inherited from block input  x0=0  Ts=Ts
  Vg : Outport
  wires:
  u/1 -> Lead-Lag (Discrete or Continuous)/1
  Lead-Lag (Discrete or Continuous)/1 -> Vg/1

== system DataCenterStability/UPS/Inverter/Filter & Measurements/ Measurements/Measurement2 ==
  u : Inport
  Lead-Lag (Discrete or Continuous) : eeGeneralControl/Lead-Lag (Discrete or Continuous)  T1=0  T2=1e-3  B=inf  A=-inf  init_option=Inherited from block input  x0=0  Ts=Ts
  Vg : Outport
  wires:
  u/1 -> Lead-Lag (Discrete or Continuous)/1
  Lead-Lag (Discrete or Continuous)/1 -> Vg/1

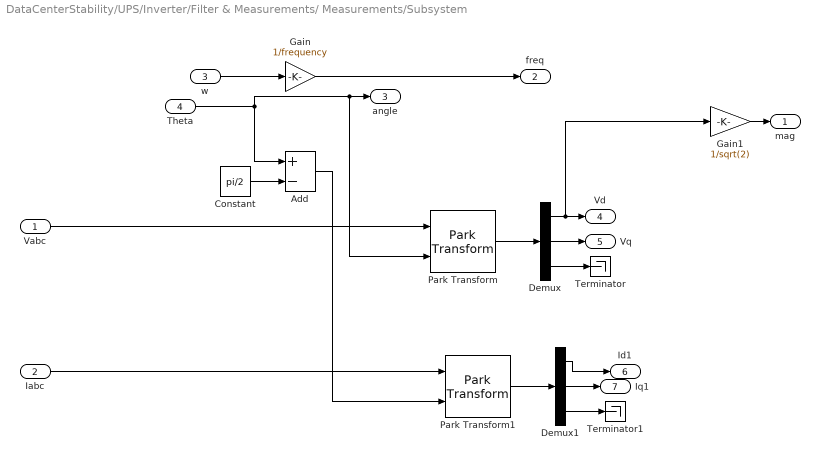
== system DataCenterStability/UPS/Inverter/Filter & Measurements/ Measurements/Subsystem ==
  Vabc : Inport
  Iabc : Inport  Port=2
  w : Inport  Port=3
  Theta : Inport  Port=4
  Add : Sum  Inputs=+-
  Constant : Constant  Value=pi/2
  Demux : Demux  Outputs=3
  Demux1 : Demux  Outputs=3
  Gain : Gain  Gain=1/frequency
  Gain1 : Gain  Gain=1/sqrt(2)
  Park Transform : eeTransforms/Park Transform  AxisAlignment=Q-axis  PowerInvariant=off
  Park Transform1 : eeTransforms/Park Transform  AxisAlignment=D-axis  PowerInvariant=off
  Terminator : Terminator
  Terminator1 : Terminator
  mag : Outport
  freq : Outport  Port=2
  angle : Outport  Port=3
  Vd : Outport  Port=4
  Vq : Outport  Port=5
  Id1 : Outport  Port=6
  Iq1 : Outport  Port=7
  wires:
  Iabc/1 -> Park Transform1/1
  Demux1/3 -> Terminator1/1
  Demux1/2 -> Iq1/1
  Demux1/1 -> Id1/1
  Park Transform1/1 -> Demux1/1
  w/1 -> Gain/1
  Theta/1 -> Park Transform/2, angle/1, Add/1
  Demux/2 -> Vq/1
  Demux/1 -> Gain1/1, Vd/1
  Park Transform/1 -> Demux/1
  Vabc/1 -> Park Transform/1
  Demux/3 -> Terminator/1
  Gain/1 -> freq/1
  Gain1/1 -> mag/1
  Constant/1 -> Add/2
  Add/1 -> Park Transform1/2

== system DataCenterStability/UPS/Inverter/Inverter Controller/Current Limiter/Current Limiter ==
  Igd : Inport
  Igq : Inport  Port=2
  Current Saturation : Subsystem  VariantControl=Current Saturation
  Virtual Impedance : Subsystem  VariantControl=Virtual Impedance
  delVd : Outport
  delVq : Outport  Port=2
  Idmax : Outport  Port=3
  Iqmax : Outport  Port=4

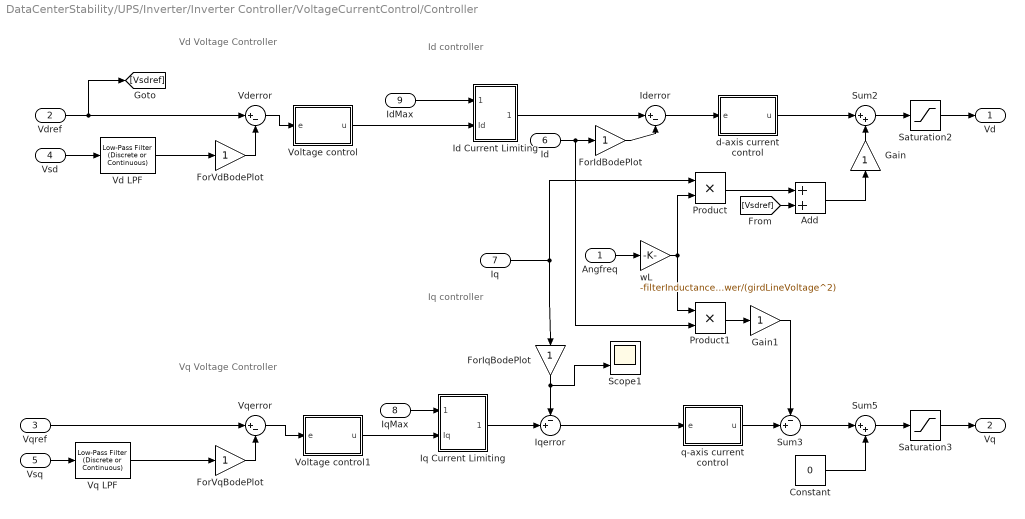
== system DataCenterStability/UPS/Inverter/Inverter Controller/VoltageCurrentControl/Controller ==
  note: Vq Voltage Controller
  note: Iq controller
  note: Vd Voltage Controller
  note: Id controller
  Angfreq : Inport
  Vdref : Inport  Port=2
  Vqref : Inport  Port=3
  Vsd : Inport  Port=4
  Vsq : Inport  Port=5
  Id : Inport  Port=6
  Iq : Inport  Port=7
  IqMax : Inport  Port=8
  IdMax : Inport  Port=9
  Add : Sum
  Constant : Constant  Value=0  SampleTime=currentControlTs
  ForIdBodePlot : Gain
  ForIqBodePlot : Gain
  ForVdBodePlot : Gain
  ForVqBodePlot : Gain
  Gain : Gain
  Gain1 : Gain
  Id Current Limiting : Subsystem
  Iderror : Sum  Inputs=|+-
  Iq Current Limiting : Subsystem
  Iqerror : Sum  Inputs=-+|
  Product : Product
  Product1 : Product
  Saturation2 : Saturate  UpperLimit=1.5  LowerLimit=-1.5
  Saturation3 : Saturate  UpperLimit=1.5  LowerLimit=-1.5
  Scope1 : Scope  NumInputPorts=2
      settings: ActiveDisplayYMinimum=-0.5206159009733754  ActiveDisplayYMaximum=0.33911481242712255
  Sum2 : Sum  Inputs=|++
  Sum3 : Sum  Inputs=-+|
  Sum5 : Sum  Inputs=|++
  Vd LPF : eeGeneralControl/Low-Pass Filter (Discrete or Continuous)  K=1  T=vdvqLPFTimeConst  B=inf  A=-inf  init_option=Specify as parameter  x0=0  Ts=voltControlTs
  Vderror : Sum  Inputs=|+-
  Voltage control : Subsystem
  Voltage control1 : Subsystem
  Vq LPF : eeGeneralControl/Low-Pass Filter (Discrete or Continuous)  K=1  T=vdvqLPFTimeConst  B=inf  A=-inf  init_option=Inherited from block input  x0=0  Ts=voltControlTs
  Vqerror : Sum  Inputs=|+-
  d-axis current control : Subsystem
  q-axis current control : Subsystem
  wL : Gain  Gain=-filterInductance*power/(girdLineVoltage^2)
  Vd : Outport  VectorParamsAs1DForOutWhenUnconnected=off
  Vq : Outport  Port=2  VectorParamsAs1DForOutWhenUnconnected=off
  wires:
  Vdref/1 -> [Vsdref], Vderror/1
  Vq LPF/1 -> ForVqBodePlot/1
  Vd LPF/1 -> ForVdBodePlot/1
  ForIqBodePlot/1 -> Iqerror/1, Scope1/2
  ForIdBodePlot/1 -> Iderror/2
  ForVqBodePlot/1 -> Vqerror/2
  ForVdBodePlot/1 -> Vderror/2
  Vsd/1 -> Vd LPF/1
  Gain/1 -> Sum2/2
  Add/1 -> Gain/1
  [Vsdref] -> Add/2
  Gain1/1 -> Sum3/1
  Vqerror/1 -> Voltage control1/1(e)
  Vqref/1 -> Vqerror/1
  Vderror/1 -> Voltage control/1(e)
  Id/1 -> ForIdBodePlot/1, Product1/2
  Vsq/1 -> Vq LPF/1
  Sum5/1 -> Saturation3/1
  Sum3/1 -> Sum5/1
  q-axis current control/1(u) -> Sum3/2
  Sum2/1 -> Saturation2/1
  d-axis current control/1(u) -> Sum2/1
  Product/1 -> Add/1
  Product1/1 -> Gain1/1
  Saturation2/1 -> Vd/1
  Saturation3/1 -> Vq/1
  Iderror/1 -> d-axis current control/1(e)
  Constant/1 -> Sum5/2
  Angfreq/1 -> wL/1
  wL/1 -> Product/2, Product1/1
  Iqerror/1 -> q-axis current control/1(e)
  Iq/1 -> Product/1, ForIqBodePlot/1
  IdMax/1 -> Id Current Limiting/1(Imax)
  IqMax/1 -> Iq Current Limiting/1(Imax)
  Voltage control/1(u) -> Id Current Limiting/2(Id)
  Id Current Limiting/1(Idref) -> Iderror/1
  Voltage control1/1(u) -> Iq Current Limiting/2(Iq)
  Iq Current Limiting/1(Iqref) -> Iqerror/2

== system DataCenterStability/UPS/Inverter/Inverter Controller/VoltageCurrentControl/Modulation Signal ==
  Vd : Inport
  Vq : Inport  Port=2
  Angle : Inport  Port=3
  Constant : Constant  Value=0
  Inverse Park Transform : eeTransforms/Inverse Park Transform  AxisAlignment=D-axis  PowerInvariant=off
  Mux1 : Mux  Inputs=3
  Saturation : Saturate  UpperLimit=1.2  LowerLimit=-1.2
  Saturation1 : Saturate
  Saturation2 : Saturate  UpperLimit=1  LowerLimit=-1
  mabc : Outport  VectorParamsAs1DForOutWhenUnconnected=off
  wires:
  Vq/1 -> Saturation1/1
  Vd/1 -> Saturation/1
  Constant/1 -> Mux1/3
  Saturation2/1 -> mabc/1
  Angle/1 -> Inverse Park Transform/2
  Mux1/1 -> Inverse Park Transform/1
  Inverse Park Transform/1 -> Saturation2/1
  Saturation/1 -> Mux1/1
  Saturation1/1 -> Mux1/2

== system DataCenterStability/UPS/Rectifier/PFC Rectifier Controller/Current Controller/Id and Iq Controller ==
  idRef : Inport
  iqRef : Inport  Port=2
  IdSens : Inport  Port=3
  iqSens : Inport  Port=4
  vd : Inport  Port=5
  vq : Inport  Port=6
  Reset : Inport  Port=7
  Constant4 : Constant  Value=0  SampleTime=Ts
  Gain1 : Gain  Gain=2*1*pi*Freq*L/BaseImpedance
  Gain2 : Gain  Gain=2*1*pi*Freq*L/BaseImpedance
  IdPID : slpidlib/PID Controller  Controller=PID  Form=Parallel  TimeDomain=Discrete-time  UseExternalTs=off  SampleTime=Ts  IntegratorMethod=Forward Euler  FilterMethod=Forward Euler  ControllerParametersSource=internal  P=KpdCurrent  I=KidCurrent  UseKiTs=off  D=KddCurrent  UseExternalDerivativeSource=off  N=NdCurrent  UseFilter=on  TunerSelectOption=Transfer Function Based (PID Tuner App)  InitialConditionSource=internal  InitialConditionForIntegrator=0  InitialConditionForFilter=0  DifferentiatorICPrevScaledInput=0  ExternalReset=falling  TrackingMode=off  Kt=1  LimitOutput=on  SatLimitsSource=internal  UpperSaturationLimit=IdControlUpperLimit  LowerSaturationLimit=IdControlLowerLimit  LinearizeAsGain=on  AntiWindupMode=clamping  Kb=1  LimitIntegrator=on  UpperIntegratorSaturationLimit=IdControlUpperLimit  LowerIntegratorSaturationLimit=IdControlLowerLimit  POutMin=[]  POutMax=[]  IOutMin=[]  IOutMax=[]  DOutMin=[]  DOutMax=[]  NOutMin=[]  NOutMax=[]  SumOutMin=[]  SumOutMax=[]  SaturationOutMin=[]  SaturationOutMax=[]  PParamMin=[]  PParamMax=[]  IParamMin=[]  IParamMax=[]  DParamMin=[]  DParamMax=[]  NParamMin=[]  NParamMax=[]  KbParamMin=[]  KbParamMax=[]  KtParamMin=[]  KtParamMax=[]  KbOutMin=[]  KbOutMax=[]  KtOutMin=[]  KtOutMax=[]  IntegratorOutMin=[]  IntegratorOutMax=[]  FilterOutMin=[]  FilterOutMax=[]  SumI1OutMin=[]  SumI1OutMax=[]  SumI2OutMin=[]  SumI2OutMax=[]  SumI3OutMin=[]  SumI3OutMax=[]  SumI4OutMin=[]  SumI4OutMax=[]  SumDOutMin=[]  SumDOutMax=[]  DifferentiatorOutMin=[]  DifferentiatorOutMax=[]  FilterDiffOutCoefMin=[]  FilterDiffOutCoefMax=[]  ReciprocalOutMin=[]  ReciprocalOutMax=[]  SumDenOutMin=[]  SumDenOutMax=[]  SumNumOutMin=[]  SumNumOutMax=[]  DivideOutMin=[]  DivideOutMax=[]  UdiffTsProdOutMin=[]  UdiffTsProdOutMax=[]  NTsProdOutMin=[]  NTsProdOutMax=[]  UintegralTsProdOutMin=[]  UintegralTsProdOutMax=[]  UngainTsProdOutMin=[]  UngainTsProdOutMax=[]  ClampingZeroOutDataTypeStr=Inherit: Inherit via back propagation  ClampingZeroOutMin=[]  ClampingZeroOutMax=[]  FilterDenConstantOutDataTypeStr=Inherit: Inherit via back propagation  FilterDenConstantOutMin=[]  FilterDenConstantOutMax=[]  PCopyOutDataTypeStr=Inherit: Inherit via back propagation  PCopyOutMin=[]  PCopyOutMax=[]  NCopyOutDataTypeStr=Inherit: Inherit via back propagation  NCopyOutMin=[]  NCopyOutMax=[]  IntegratorContinuousStateAttributes=''  IntegratorStateMustResolveToSignalObject=off  IntegratorRTWStateStorageClass=Auto  FilterContinuousStateAttributes=''  FilterStateMustResolveToSignalObject=off  FilterRTWStateStorageClass=Auto  ParallelPVariant=InternalParameters  IdealPVariant=Disabled  IVariant=InternalParameters  DVariant=InternalParameters  IntegratorVariant=Discrete  SatVariant=Enabled  AWVariant=DiscClampingParallel  PCopyVariant=Disabled  TRVariant=Disabled  FdbkBlocksVariant=Forward  IdealPFdbkVariant=Disabled  SatFdbkVariant=Disabled  DerivativeFilterVariant=ForwardEulerFilter  NVariant=InternalParameters  NCopyVariant=Disabled  FilterICVariant=InternalICsFilter  IntegratorICVariant=InternalICs  ExternalResetVariant=ExternalReset  TRSumVariant=Passthrough  SumFdbkVariant=Disabled  SumVariant=Sum_PID  TsampFilterVariant=InternalTs  TsampNgainVariant=Passthrough  TsampIntegralVariant=Disabled_SignalSpec  ExternalSaturationOutDataTypeStr=Inherit: Same as second input  DerivativeSourceVariant=ErrorSignal  PreIntVariant=InternalPreInt
  IqPID : slpidlib/PID Controller  Controller=PID  Form=Parallel  TimeDomain=Discrete-time  UseExternalTs=off  SampleTime=Ts  IntegratorMethod=Forward Euler  FilterMethod=Forward Euler  ControllerParametersSource=internal  P=KpqCurrent  I=KiqCurrent  UseKiTs=off  D=KdqCurrent  UseExternalDerivativeSource=off  N=NdCurrent  UseFilter=on  TunerSelectOption=Transfer Function Based (PID Tuner App)  InitialConditionSource=internal  InitialConditionForIntegrator=0  InitialConditionForFilter=0  DifferentiatorICPrevScaledInput=0  ExternalReset=falling  TrackingMode=off  Kt=1  LimitOutput=on  SatLimitsSource=internal  UpperSaturationLimit=IqControlUpperLimit  LowerSaturationLimit=IqControlLowerLimit  LinearizeAsGain=on  AntiWindupMode=clamping  Kb=1  LimitIntegrator=on  UpperIntegratorSaturationLimit=IqControlUpperLimit  LowerIntegratorSaturationLimit=IqControlLowerLimit  POutMin=[]  POutMax=[]  IOutMin=[]  IOutMax=[]  DOutMin=[]  DOutMax=[]  NOutMin=[]  NOutMax=[]  SumOutMin=[]  SumOutMax=[]  SaturationOutMin=[]  SaturationOutMax=[]  PParamMin=[]  PParamMax=[]  IParamMin=[]  IParamMax=[]  DParamMin=[]  DParamMax=[]  NParamMin=[]  NParamMax=[]  KbParamMin=[]  KbParamMax=[]  KtParamMin=[]  KtParamMax=[]  KbOutMin=[]  KbOutMax=[]  KtOutMin=[]  KtOutMax=[]  IntegratorOutMin=[]  IntegratorOutMax=[]  FilterOutMin=[]  FilterOutMax=[]  SumI1OutMin=[]  SumI1OutMax=[]  SumI2OutMin=[]  SumI2OutMax=[]  SumI3OutMin=[]  SumI3OutMax=[]  SumI4OutMin=[]  SumI4OutMax=[]  SumDOutMin=[]  SumDOutMax=[]  DifferentiatorOutMin=[]  DifferentiatorOutMax=[]  FilterDiffOutCoefMin=[]  FilterDiffOutCoefMax=[]  ReciprocalOutMin=[]  ReciprocalOutMax=[]  SumDenOutMin=[]  SumDenOutMax=[]  SumNumOutMin=[]  SumNumOutMax=[]  DivideOutMin=[]  DivideOutMax=[]  UdiffTsProdOutMin=[]  UdiffTsProdOutMax=[]  NTsProdOutMin=[]  NTsProdOutMax=[]  UintegralTsProdOutMin=[]  UintegralTsProdOutMax=[]  UngainTsProdOutMin=[]  UngainTsProdOutMax=[]  ClampingZeroOutDataTypeStr=Inherit: Inherit via back propagation  ClampingZeroOutMin=[]  ClampingZeroOutMax=[]  FilterDenConstantOutDataTypeStr=Inherit: Inherit via back propagation  FilterDenConstantOutMin=[]  FilterDenConstantOutMax=[]  PCopyOutDataTypeStr=Inherit: Inherit via back propagation  PCopyOutMin=[]  PCopyOutMax=[]  NCopyOutDataTypeStr=Inherit: Inherit via back propagation  NCopyOutMin=[]  NCopyOutMax=[]  IntegratorContinuousStateAttributes=''  IntegratorStateMustResolveToSignalObject=off  IntegratorRTWStateStorageClass=Auto  FilterContinuousStateAttributes=''  FilterStateMustResolveToSignalObject=off  FilterRTWStateStorageClass=Auto  ParallelPVariant=InternalParameters  IdealPVariant=Disabled  IVariant=InternalParameters  DVariant=InternalParameters  IntegratorVariant=Discrete  SatVariant=Enabled  AWVariant=DiscClampingParallel  PCopyVariant=Disabled  TRVariant=Disabled  FdbkBlocksVariant=Forward  IdealPFdbkVariant=Disabled  SatFdbkVariant=Disabled  DerivativeFilterVariant=ForwardEulerFilter  NVariant=InternalParameters  NCopyVariant=Disabled  FilterICVariant=InternalICsFilter  IntegratorICVariant=InternalICs  ExternalResetVariant=ExternalReset  TRSumVariant=Passthrough  SumFdbkVariant=Disabled  SumVariant=Sum_PID  TsampFilterVariant=InternalTs  TsampNgainVariant=Passthrough  TsampIntegralVariant=Disabled_SignalSpec  ExternalSaturationOutDataTypeStr=Inherit: Same as second input  DerivativeSourceVariant=ErrorSignal  PreIntVariant=InternalPreInt
  Mux1 : Mux  Inputs=3
  Sum1 : Sum  Inputs=|+-
  Sum2 : Sum  Inputs=|+-+
  Sum4 : Sum  Inputs=|--+
  Sum5 : Sum  Inputs=|+-
  vdqoRef : Outport
  IdCntrlError : Outport  Port=2
  IqCntrlError : Outport  Port=3
  wires:
  iqRef/1 -> Sum5/1
  Mux1/1 -> vdqoRef/1
  idRef/1 -> Sum1/1
  IqPID/1 -> Sum4/2
  IdSens/1 -> Gain1/1, Sum1/2
  Sum1/1 -> IdPID/1, IdCntrlError/1
  vd/1 -> Sum2/1
  IdPID/1 -> Sum2/2
  Gain2/1 -> Sum2/3
  Gain1/1 -> Sum4/1
  vq/1 -> Sum4/3
  iqSens/1 -> Gain2/1, Sum5/2
  Sum2/1 -> Mux1/1
  Sum4/1 -> Mux1/2
  Sum5/1 -> IqPID/1, IqCntrlError/1
  Constant4/1 -> Mux1/3
  Reset/1 -> IqPID/2, IdPID/2

== system DataCenterStability/UPS/Rectifier/PFC Rectifier Controller/DC Voltage Controller and Current Reference/Iq Reference ==
  V_mag : Inport
  Q_ref : Inport  Port=2
  Divide2 : Product  Inputs=*/
  iq_ref : Outport
  wires:
  V_mag/1 -> Divide2/2
  Q_ref/1 -> Divide2/1
  Divide2/1 -> iq_ref/1

== system DataCenterStability/UPS/Rectifier/PFC Rectifier Controller/DC Voltage Controller and Current Reference/Voltage Controller ==
  Vdcref : Inport
  Vdcmeas : Inport  Port=2
  Reset : Inport  Port=3
  Gain : Gain  Gain=1/BaseVdc
  Saturation : Saturate  UpperLimit=1.5  LowerLimit=0
  Sum : Sum  Inputs=|+-
  Voltage control : Subsystem
  Id : Outport
  wires:
  Sum/1 -> Gain/1
  Gain/1 -> Voltage control/1(e)
  Vdcmeas/1 -> Sum/2
  Vdcref/1 -> Sum/1
  Voltage control/1(u) -> Saturation/1
  Saturation/1 -> Id/1
  Reset/1 -> Voltage control/2(Reset)

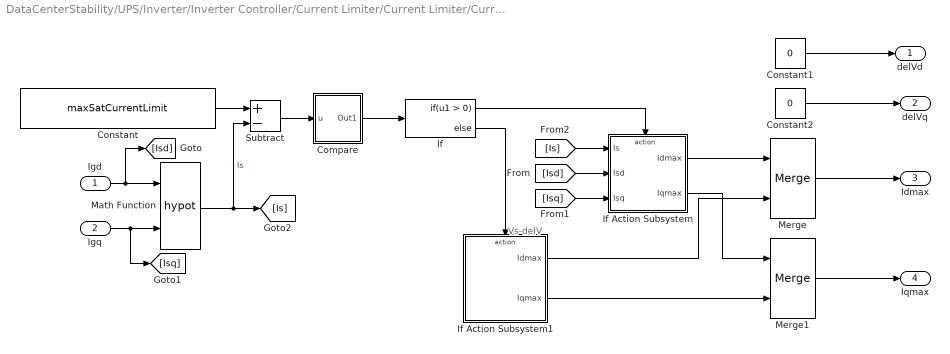
== system DataCenterStability/UPS/Inverter/Inverter Controller/Current Limiter/Current Limiter/Current Saturation ==
  note: Vs-delV
  Igd : Inport
  Igq : Inport  Port=2
  Compare : Subsystem
  Constant : Constant  Value=maxSatCurrentLimit
  Constant1 : Constant  Value=0
  Constant2 : Constant  Value=0
  If : If
  If Action Subsystem : Subsystem  TreatAsAtomicUnit=on
  If Action Subsystem1 : Subsystem  TreatAsAtomicUnit=on
  Math Function : Math  Operator=hypot
  Merge : Merge
  Merge1 : Merge
  Subtract : Sum  Inputs=+-
  delVd : Outport
  delVq : Outport  Port=2
  Idmax : Outport  Port=3
  Iqmax : Outport  Port=4
  wires:
  Igd/1 -> [Isd], Math Function/1
  Igq/1 -> [Isq], Math Function/2
  Constant/1 -> Subtract/1
  Math Function/1 -> [Is], Subtract/2  "Is"
  If/1 -> If Action Subsystem/Action
  [Isd] -> If Action Subsystem/2(Isd)
  [Isq] -> If Action Subsystem/3(Isq)
  Subtract/1 -> Compare/1(u)
  Compare/1(Out1) -> If/1
  If/2 -> If Action Subsystem1/Action
  [Is] -> If Action Subsystem/1(Is)
  If Action Subsystem/1(Idmax) -> Merge/1
  If Action Subsystem1/1(Idmax) -> Merge/2
  If Action Subsystem/2(Iqmax) -> Merge1/1
  If Action Subsystem1/2(Iqmax) -> Merge1/2
  Constant2/1 -> delVq/1
  Constant1/1 -> delVd/1
  Merge/1 -> Idmax/1
  Merge1/1 -> Iqmax/1
